simulink model "vehicleDynamics"  (R2020a)
settings: Solver=VariableStepAuto  StartTime=0.0  StopTime=1588431736.7  RelTol=1e-3
model workspace (MAT data in the model file):
  SDO_OutputTimes = [1588431297.25 1588431297.3 1588431297.35 1588431297.4 1588431297.45 1588431297.5 1588431297.55 1588431297.6 1588431297.65 1588431297.7 1588431297.75 1588431297.8 ... (8790 elements, 8790x1)]
undefined symbols (not defined in the file): adc, g, KE, KT, L, m, magnitude, MFT, R, ra, rrc, vwc
(part 1 of 2)
settings Model: OrderedModelArguments=off  Creator=Lin  LastModifiedBy=Lin
settings DataIOCC: ExternalInput=tp820cf435_4294_44b4_a9a0_f8f238c8385d(1)  LoadExternalInput=on  OutputOption=AdditionalOutputTimes  OutputTimes=SDO_OutputTimes  ReturnWorkspaceOutputsName=SDOSimTest_Log

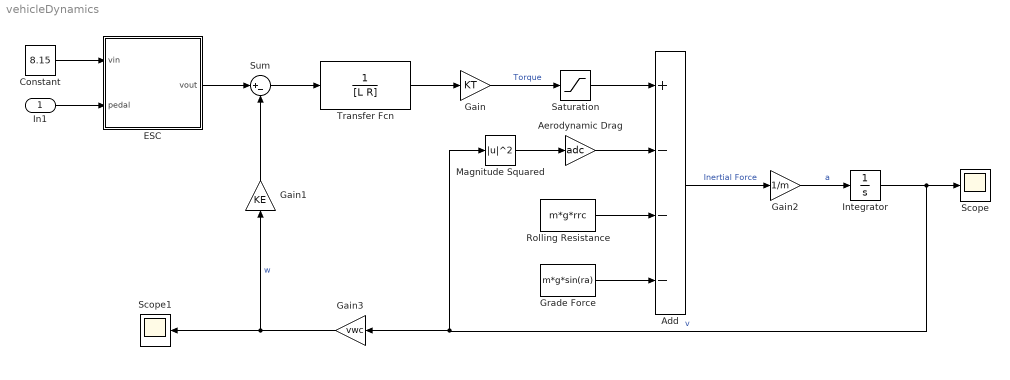
== system vehicleDynamics ==
  In1 : Inport
  Add : Sum  Inputs=+---
  Aerodynamic Drag : Gain  Gain=adc
  Constant : Constant  Value=8.15  OutMin=-1  OutMax=9
  ESC : MATLAB Function  TreatAsAtomicUnit=on
  Gain : Gain  Gain=KT
  Gain1 : Gain  Gain=KE
  Gain2 : Gain  Gain=1/m
  Gain3 : Gain  Gain=vwc
  Grade Force : Constant  Value=m*g*sin(ra)
  Integrator : Integrator
  Magnitude Squared : Math  Operator=magnitude^2  SaturateOnIntegerOverflow=on
  Rolling Resistance : Constant  Value=m*g*rrc
  Saturation : Saturate  UpperLimit=MFT  LowerLimit=-MFT
  Scope : Scope
  Scope1 : Scope
  Sum : Sum  Inputs=|+-
  Transfer Fcn : TransferFcn  Denominator=[L R]
  wires:
  Constant/1 -> ESC/1(vin)
  ESC/1(vout) -> Sum/1
  Gain1/1 -> Sum/2
  Sum/1 -> Transfer Fcn/1
  Transfer Fcn/1 -> Gain/1
  Gain/1 -> Saturation/1  "Torque"
  Rolling Resistance/1 -> Add/3
  Grade Force/1 -> Add/4
  Aerodynamic Drag/1 -> Add/2
  Magnitude Squared/1 -> Aerodynamic Drag/1
  Add/1 -> Gain2/1  "Inertial Force"
  Gain2/1 -> Integrator/1  "a"
  Integrator/1 -> Gain3/1, Magnitude Squared/1, Scope/1  "v"
  Gain3/1 -> Scope1/1, Gain1/1  "w"
  Saturation/1 -> Add/1
  In1/1 -> ESC/2(pedal)
